simulink model "updated_cell_model"  (R2023a)
settings: Solver=VariableStepAuto  StartTime=0.0  StopTime=T_e  RelTol=1e-3
libraries: nesl_utility x9, fl_lib x8, BatteryEstimators x1, ee_lib x1, spspowerguiLib x1
settings Model: Creator=Lenovo  LastModifiedBy=Lenovo

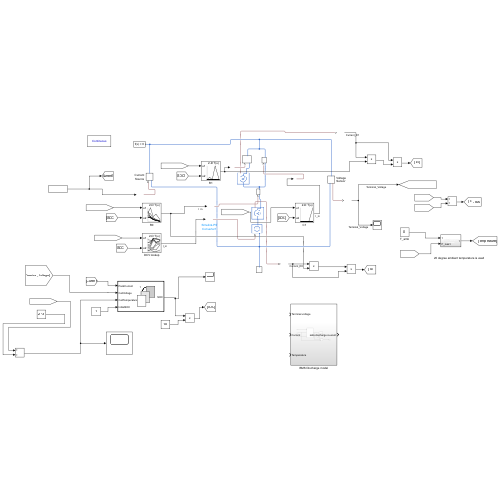
[thumbnail: Simulink's stored preview of the top-level diagram]
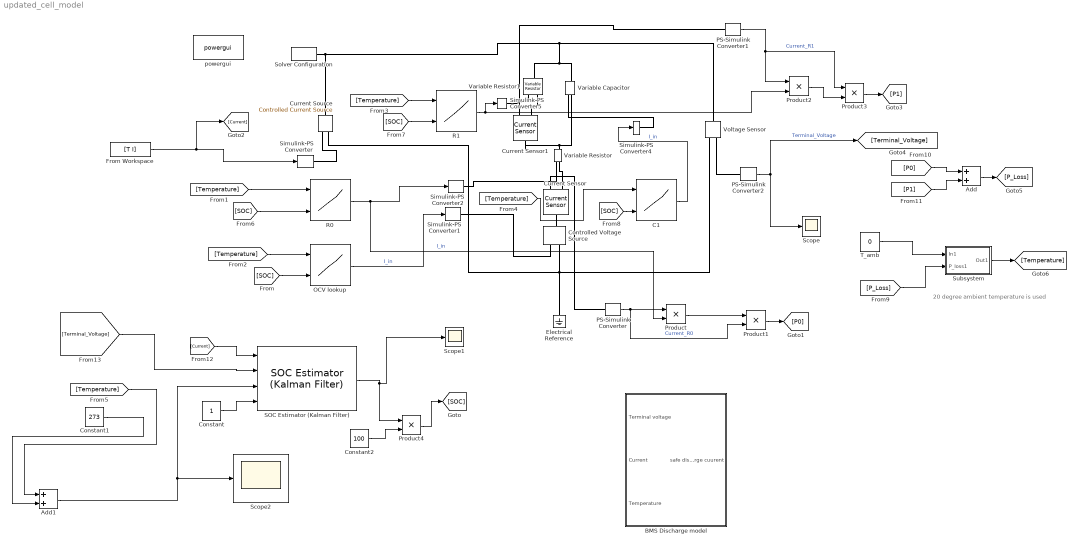
== system updated_cell_model ==
  note: 20 degree ambient temperature is used
  Add : Sum
  Add1 : Sum
  BMS Discharge model : Subsystem
  C1 : Lookup_n-D  BreakpointsForDimension1=[-20;-10;0;10;25]  BreakpointsForDimension2=[10;20;30;40;50;60;70;80;90;100]  Table=[16 15.6 21.9 12.1 12.5 14.6 13.6 24.3 273.7 8.7;297.5197 90.758 403.5264 495.9754 857.8368 533.7226 962.1347 33.0545 927.6445 6.7778;25.1 123.5 1235.4 1047 4719.7 2413 3586.7 1727.4 2526.3 2511.9;460.7201 3493.6 4723.4 2574.8 8517.3 4491.2 1813.7 2264.8 3365.1 2995.5;2468.8 6800.2 4626.1 934790 7336.3 3942.9 4597.4 3716.8 4825 4798.6]  InternalRulePriority=Speed  RndMeth=Simplest
      settings: InputPortMap=u0,u1
  Constant : Constant
  Constant1 : Constant  Value=273
  Constant2 : Constant  Value=100
  Controlled Voltage Source : fl_lib/Electrical/Electrical Sources/Controlled Voltage Source
  Current Source : fl_lib/Electrical/Electrical Sources/Controlled Current Source
  Current Sensor : fl_lib/Electrical/Electrical Sensors/Current Sensor
  Current Sensor1 : fl_lib/Electrical/Electrical Sensors/Current Sensor
  Electrical Reference : fl_lib/Electrical/Electrical Elements/Electrical Reference
  From Workspace : FromWorkspace  VariableName=[T I]
  OCV lookup : Lookup_n-D  BreakpointsForDimension1=[-20;-10;0;10;25]  BreakpointsForDimension2=[10;20;30;40;50;60;70;80;90;100]  Table=[3.4 3.4133 3.512 3.5847 3.6579 3.76 3.8253 3.9741 3.98 4.1415;3.4586 3.446 3.5449 3.6079 3.684 3.7768 3.8732 3.9371 4.0233 4.1351;3.3426 3.4651 3.552 3.6089 4.0935 4.2271 4.2269 4.2754 4.2364 4.1297;3.3288 3.4524 3.7717 3.8828 3.9466 3.9889 3.9711 4.236 4.2233 4.1442;3.4449 3.8033 3.8678 3.9402 4.0192 4.0839 4.0834 4.1074 4.1817 4.1705]  InternalRulePriority=Speed  RndMeth=Simplest
      settings: InputPortMap=u0,u1
  PS-Simulink Converter : nesl_utility/PS-Simulink Converter  PhysicalDomain=network_engine_domain  SubClassName=ps_output  LeftPortType=input  RightPortType=output  PseudoPeriodic=off  Frequencies=[]  VectorFormat=1-D array  Unit=A  AffineConversion=off
  PS-Simulink Converter1 : nesl_utility/PS-Simulink Converter  PhysicalDomain=network_engine_domain  SubClassName=ps_output  LeftPortType=input  RightPortType=output  PseudoPeriodic=off  Frequencies=[]  VectorFormat=1-D array  Unit=A  AffineConversion=off
  PS-Simulink Converter2 : nesl_utility/PS-Simulink Converter  PhysicalDomain=network_engine_domain  SubClassName=ps_output  LeftPortType=input  RightPortType=output  PseudoPeriodic=off  Frequencies=[]  VectorFormat=1-D array  Unit=V  AffineConversion=off
  Product{,1..4} (5 alike) : Product
  R0 : Lookup_n-D  BreakpointsForDimension1=[-20;-10;0;10;25]  BreakpointsForDimension2=[10;20;30;40;50;60;70;80;90;100]  Table=[0.17 0.1669 0.122 0.0987 0.0946 0.0989 0.098 0.125 0.1909 0.1531;0.2465 0.1484 0.104 0.0887 0.09 0.0881 0.0896 0.086 0.1 0.1041;0.1094 0.0856 0.0649 0.0617 0.062 0.0612 0.0621 0.0659 0.0682 0.0867;0.1447 0.0603 0.046 0.0454 0.0447 0.0453 0.0467 0.049 0.0492 0.0644;0.0604 0.0357 0.0343 0.0326 0.0326 0.0327 0.0367 0.032 0.0347 0.0417]  InternalRulePriority=Speed  RndMeth=Simplest
      settings: InputPortMap=u0,u1
  R1 : Lookup_n-D  BreakpointsForDimension1=[-20;-10;0;10;25]  BreakpointsForDimension2=[10;20;30;40;50;60;70;80;90;100]  Table=[0.37 0.3742 0.1134 0.0845 0.083 0.0828 0.0742 0.0988 0.0324 0.1693;3766.9 0.0894 0.033 0.022 0.0706 0.0462 0.0548 0.0732 0.0418 0.072;0.2602 0.0384 0.0488 0.0037 2.2412 10.5216 15.2602 8.7746 13.8938 0.0068;0.8416 0.1226 2.3076 3.94 9.5012 22206 0.2322 3.9946 14.149 0.7259;1.0244 2.5685 9.784 0.4363 4.4983 16.0326 13.3701 9.6224 0.9478 17.7687]  InternalRulePriority=Speed  RndMeth=Simplest
      settings: InputPortMap=u0,u1
  SOC Estimator (Kalman Filter) : BatteryEstimators/SOC Estimator (Kalman Filter)  filterType=Unscented Kalman-Bucy filter  alpha=1  beta=2  kappa=0  Q=|  R=0.1  P0=[1e-5 0; 0 1]  Ts=1  SOC_vec=[.1, .2, .3, .4, .5, .6, .7, .8 , .9, 1]  T_vec=[253, 263, 273, 283, 298]  R0_mat=R0_SOC  R1_mat=R1_SOC  tau1_mat=tau1_SOC  V0_mat=OCV_SOC  AH=2.9
      | [1e-6 0;
      | 0 1e-6]
      settings: LibrarySourceBlock=|
      | batt_sl_lib/Estimators/SOC Estimator
      | (Kalman Filter)
  Scope : Scope
  Scope1 : Scope
  Scope2 : Scope
  Simulink-PS Converter : nesl_utility/Simulink-PS Converter  PhysicalDomain=network_engine_domain  SubClassName=ps_input  LeftPortType=input  RightPortType=output  PseudoPeriodic=off  Frequencies=[]  NoiseDistribution=none  NoiseParameters=[]  Unit=A  AffineConversion=off  FilteringAndDerivatives=zero  SimscapeFilterOrder=1  InputFilterTimeConstant=.001  UdotUserProvided=0
  Simulink-PS Converter1 : nesl_utility/Simulink-PS Converter  PhysicalDomain=network_engine_domain  SubClassName=ps_input  LeftPortType=input  RightPortType=output  PseudoPeriodic=off  Frequencies=[]  NoiseDistribution=none  NoiseParameters=[]  Unit=V  AffineConversion=off  FilteringAndDerivatives=zero  SimscapeFilterOrder=1  InputFilterTimeConstant=.001  UdotUserProvided=0
  Simulink-PS Converter2 : nesl_utility/Simulink-PS Converter  PhysicalDomain=network_engine_domain  SubClassName=ps_input  LeftPortType=input  RightPortType=output  PseudoPeriodic=off  Frequencies=[]  NoiseDistribution=none  NoiseParameters=[]  Unit=Ohm  AffineConversion=off  FilteringAndDerivatives=zero  SimscapeFilterOrder=1  InputFilterTimeConstant=.001  UdotUserProvided=0
  Simulink-PS Converter4 : nesl_utility/Simulink-PS Converter  PhysicalDomain=network_engine_domain  SubClassName=ps_input  LeftPortType=input  RightPortType=output  PseudoPeriodic=off  Frequencies=[]  NoiseDistribution=none  NoiseParameters=[]  Unit=F  AffineConversion=off  FilteringAndDerivatives=zero  SimscapeFilterOrder=1  InputFilterTimeConstant=.001  UdotUserProvided=0
  Simulink-PS Converter5 : nesl_utility/Simulink-PS Converter  PhysicalDomain=network_engine_domain  SubClassName=ps_input  LeftPortType=input  RightPortType=output  PseudoPeriodic=off  Frequencies=[]  NoiseDistribution=none  NoiseParameters=[]  Unit=Ohm  AffineConversion=on  FilteringAndDerivatives=provide  SimscapeFilterOrder=1  InputFilterTimeConstant=0.001  UdotUserProvided=0
  Solver Configuration : nesl_utility/Solver Configuration  PhysicalDomain=network_engine_domain  SubClassName=solver  LeftPortType=input  RightPortType=generic  Tones=[]  Harmonics=[]  SimulateNoise=off  Profile=off  UseLocalSampling=off  EnableSwitchedLinearOptims=on  FrequencyDomain=off  UseCCode=off  RelTol=0.001  AbsTol=1e-06  MinStep=1e-09  ToWorkspace=off  RevertToSquareIcSolve=off  NumHomotopyIterations=100  PhasorMode=off  PhasorModeNumHarmonics=1  ConsistencySolver=NEWTON_FTOL  IndexReductionMethod=DerivativeReplacement  DoDC=off  ResidualTolerance=1e-9  ConsistencyTolSource=GLOBAL  ConsistencyAbsTol=0.001  ConsistencyRelTol=0.001  ConsistencyTolFactor=0.001  UseLocalSolver=off  LocalSolverChoice=NE_BACKWARD_EULER_ADVANCER  ResolveIndetEquations=on  FunctionEvalNumThread=1  LocalSolverSampleTime=10  DoFixedCost=off  MaxNonlinIter=12  MaxModeIter=2  ComputeImpulses=off  ImpulseIterations=2  LinearAlgebra=Sparse  LinearAlgebraNumThread=0  EquationFormulation=NE_TIME_EF  DelaysMemoryBudget=1024  AutomaticFiltering=on  FilteringTimeConstant=0.001  PartitionStorageMethod=AS_NEEDED  PartitionMemoryBudget=1024  PartitionMethod=FAST
  Subsystem : Subsystem
  T_amb : Constant  Value=0
  Variable Capacitor : ee_lib/Passive/Variable Capacitor  prm=2  Cmin=1e-9 F  r=1e-6 Ohm  v0=0 V  q0=0 C
      settings: InternalSimscapePortConfiguration="{\"Bottom\":[],\"Left\":[{\"id\":\"C\",\"label\":\"C\",\"type\":\"input\"},{\"id\":\"p\",\"label\":\"+\",\"type\":\"foundation.electrical.electrical\"}],\"Right\":[{\"id\":\"n\",\"label\":\"-\",\"type\":\"foundation.electrical.electrical\"}],\"Top\":[]}"
  Variable Resistor : fl_lib/Electrical/Electrical Elements/Variable Resistor  Rmin=0 Ohm  i_specify=off  i_priority=None  i=0 A  i_nominal_specify=off  i_nominal_unit=A  i_nominal_value=1  v_specify=off  v_priority=None  v=0 V  v_nominal_specify=off  v_nominal_unit=V  v_nominal_value=1
  Variable Resistor1 : fl_lib/Electrical/Electrical Elements/Variable Resistor  Rmin=0 Ohm  i_specify=off  i_priority=None  i=0 A  i_nominal_specify=off  i_nominal_unit=A  i_nominal_value=1  v_specify=off  v_priority=None  v=0 V  v_nominal_specify=off  v_nominal_unit=V  v_nominal_value=1
  Voltage Sensor : fl_lib/Electrical/Electrical Sensors/Voltage Sensor
  powergui : spspowerguiLib/powergui  Priority=1  SimulationMode=Continuous  SampleTime=50e-6  frequency=60  Iterations=50  frequencyindice=60  Pbase=100e6  ErrMax=1e-4  UnitsV=kV  UnitsW=MW  buscounter=0  FunctionMessages=off  echomessages=off  EnableUseOfTLC=off  CurrentSourceSwitches=off  DisableSnubberDevices=off  DisableRonSwitches=off  DisableVfSwitches=off  DisplayEquations=off  AutomaticDiscreteSolvers=off  SolverType=Tustin/Backward Euler (TBE)  Interpol=off  ExternalGateDelay=off  methode=off  Ts=100  x0status=blocks  SPID=on  SwTol=0  HookPort=off  NonlinearTolerance=1e-4  nMaxIteration=100  ContinueOnMaxIteration=off  RestoreLinks=warning  ResistiveCurrentMeasurement=off  Frange=[0:2:500]  Ylog=off  Xlog=on  ShowGrid=off  save=off  variable=ZData  structure=0  ZoomFFT=off  StartTime=0.0  cycles=1  DisplayStyle=1  fundamental=60  FreqAxis=off  MaxFrequency=1000  frequencyindicesteady=1  RmsSteady=1  display=off
  wires:
  R1/1 -> Product2/2, Simulink-PS Converter5/1
  OCV lookup/1 -> Simulink-PS Converter1/1  "I_in"
  R0/1 -> Product/2, Simulink-PS Converter2/1  "I_in"
  C1/1 -> Simulink-PS Converter4/1  "I_in"
  From Workspace/1 -> [Current], Simulink-PS Converter/1
  PS-Simulink Converter/1 -> Product1/2, Product/1  "Current_R0"
  Product/1 -> Product1/1
  Product1/1 -> [P0]
  PS-Simulink Converter1/1 -> Product3/1, Product2/1  "Current_R1"
  Product2/1 -> Product3/2
  Product3/1 -> [P1]
  Add/1 -> [P_Loss]
  [P1] -> Add/2
  [P0] -> Add/1
  T_amb/1 -> Subsystem/1(In1)
  [P_Loss] -> Subsystem/2(P_loss1)
  [Temperature] -> R0/1
  [Temperature] -> OCV lookup/1
  [Temperature] -> R1/1
  [Temperature] -> C1/1
  Constant/1 -> SOC Estimator (Kalman Filter)/4
  SOC Estimator (Kalman Filter)/1 -> Product4/1, Scope1/1
  [SOC] -> OCV lookup/2
  [SOC] -> R0/2
  [SOC] -> R1/2
  [SOC] -> C1/2
  [Current] -> SOC Estimator (Kalman Filter)/1
  PS-Simulink Converter2/1 -> Scope/1, [Terminal_Voltage]  "Terminal_Voltage"
  [Terminal_Voltage] -> SOC Estimator (Kalman Filter)/2
  Subsystem/1(Out1) -> [Temperature]
  [Temperature] -> Add1/1
  Add1/1 -> SOC Estimator (Kalman Filter)/3, Scope2/1
  Constant1/1 -> Add1/2
  Constant2/1 -> Product4/2
  Product4/1 -> [SOC]
  connections:
  Solver Configuration/RConn1 -- Voltage Sensor/LConn1 -- Variable Resistor1/RConn1 -- Variable Capacitor/RConn1 -- Current Source/LConn1
  Variable Capacitor/LConn2 -- Current Sensor1/LConn1 -- Variable Resistor/RConn1
  Voltage Sensor/RConn2 -- Controlled Voltage Source/RConn2 -- Current Source/RConn2 -- Electrical Reference/LConn1
  Simulink-PS Converter2/RConn1 -- Variable Resistor/LConn1
  Simulink-PS Converter1/RConn1 -- Controlled Voltage Source/RConn1
  Simulink-PS Converter4/RConn1 -- Variable Capacitor/LConn1
  Current Source/RConn1 -- Simulink-PS Converter/RConn1
  Current Sensor/LConn1 -- Controlled Voltage Source/LConn1
  Current Sensor/RConn2 -- Variable Resistor/LConn2
  Simulink-PS Converter5/RConn1 -- Variable Resistor1/LConn1
  Current Sensor1/RConn2 -- Variable Resistor1/LConn2
  Current Sensor/RConn1 -- PS-Simulink Converter/LConn1
  Current Sensor1/RConn1 -- PS-Simulink Converter1/LConn1
  Voltage Sensor/RConn1 -- PS-Simulink Converter2/LConn1

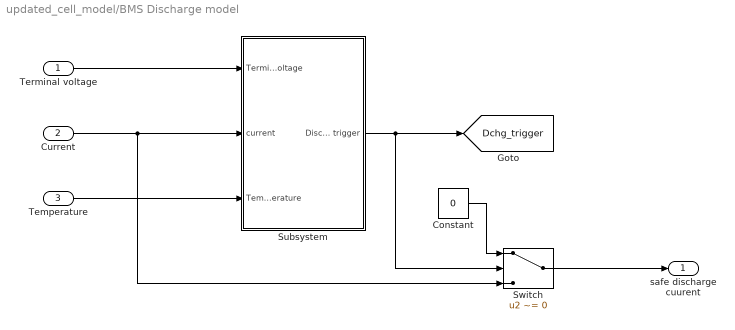
== system updated_cell_model/BMS Discharge model ==
  Terminal voltage : Inport
  Current : Inport  Port=2
  Temperature : Inport  Port=3
  Constant : Constant  Value=0
  Subsystem : Subsystem
  Switch : Switch  Criteria=u2 ~= 0  SaturateOnIntegerOverflow=off  InputSameDT=off
  safe discharge cuurent : Outport
  tag scope: Dchg_trigger=global
  wires:
  Terminal voltage/1 -> Subsystem/1(Terminal Voltage)
  Current/1 -> Switch/3, Subsystem/2(current)
  Temperature/1 -> Subsystem/3(Temperature)
  Subsystem/1(Discharge trigger) -> Switch/2, [Dchg_trigger]
  Constant/1 -> Switch/1
  Switch/1 -> safe discharge cuurent/1

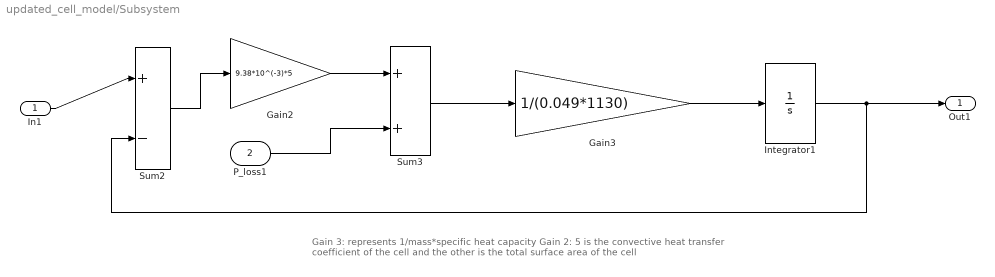
== system updated_cell_model/Subsystem ==
  note: Gain 3: represents 1/mass*specific heat capacity
      | Gain 2: 5 is the convective heat transfer coefficient of the cell and the other is the total surface area of the cell
  In1 : Inport
  P_loss1 : Inport  Port=2
  Gain2 : Gain  Gain=9.38*10^(-3)*5
  Gain3 : Gain  Gain=1/(0.049*1130)
  Integrator1 : Integrator
  Sum2 : Sum  Inputs=|+-
  Sum3 : Sum
  Out1 : Outport
  wires:
  In1/1 -> Sum2/1
  Sum3/1 -> Gain3/1
  Sum2/1 -> Gain2/1
  P_loss1/1 -> Sum3/2
  Gain3/1 -> Integrator1/1
  Integrator1/1 -> Out1/1, Sum2/2
  Gain2/1 -> Sum3/1

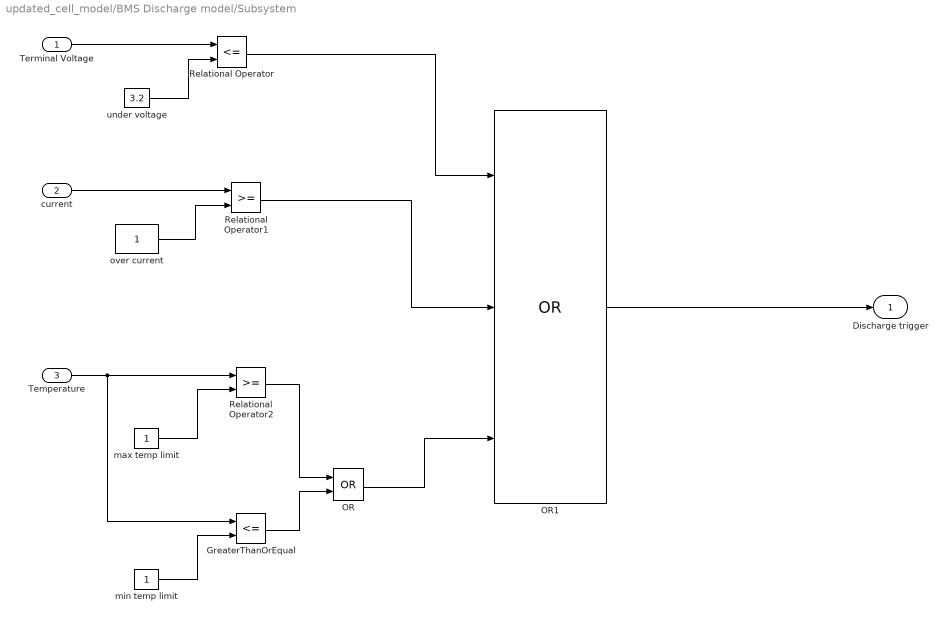
== system updated_cell_model/BMS Discharge model/Subsystem ==
  Terminal Voltage : Inport
  current : Inport  Port=2
  Temperature : Inport  Port=3
  GreaterThanOrEqual : RelationalOperator  Operator=<=  OutDataTypeStr=boolean  RndMeth=Simplest  InputSameDT=off
  OR : Logic  Operator=OR  AllPortsSameDT=off  OutDataTypeStr=boolean
  OR1 : Logic  Operator=OR  Inputs=3  AllPortsSameDT=off  OutDataTypeStr=boolean
  Relational Operator : RelationalOperator  Operator=<=  OutDataTypeStr=boolean  RndMeth=Simplest  InputSameDT=off
  Relational Operator1 : RelationalOperator  OutDataTypeStr=boolean  RndMeth=Simplest  InputSameDT=off
  Relational Operator2 : RelationalOperator  OutDataTypeStr=boolean  RndMeth=Simplest  InputSameDT=off
  max temp limit : Constant
  min temp limit : Constant
  over current : Constant
  under voltage : Constant  Value=3.2
  Discharge trigger : Outport
  wires:
  Terminal Voltage/1 -> Relational Operator/1
  under voltage/1 -> Relational Operator/2
  current/1 -> Relational Operator1/1
  over current/1 -> Relational Operator1/2
  Temperature/1 -> GreaterThanOrEqual/1, Relational Operator2/1
  max temp limit/1 -> Relational Operator2/2
  min temp limit/1 -> GreaterThanOrEqual/2
  Relational Operator2/1 -> OR/1
  GreaterThanOrEqual/1 -> OR/2
  Relational Operator/1 -> OR1/1
  Relational Operator1/1 -> OR1/2
  OR/1 -> OR1/3
  OR1/1 -> Discharge trigger/1
